simulink model "motorSimIdent"  (R2019b)
settings: Solver=VariableStepAuto  StartTime=0.0  StopTime=10.0  RelTol=1e-3
values from neighbouring files (symbols this model uses):
  b = 0.5    [MotorExpScriptIdent.m]    (also in motorSimScript.m; motorSimScriptIdent.m)
  J = 0.05    [MotorExpScriptIdent.m]    (also in motorSimScript.m; motorSimScriptIdent.m)
  K = 114.4795944    [MotorExpScriptIdent.m]    (also in motorSimScript.m = 8; motorSimScriptIdent.m = 10)
  Ke = 0.5    [MotorExpScriptIdent.m]    (also in motorSimScript.m; motorSimScriptIdent.m)
  Kt = 0.5    [MotorExpScriptIdent.m]    (also in motorSimScript.m; motorSimScriptIdent.m)
  Ra = 1    [MotorExpScriptIdent.m]    (also in motorSimScript.m; motorSimScriptIdent.m)
  sigma = 0.1147802808    [MotorExpScriptIdent.m]    (also in motorSimScript.m = 0.2; motorSimScriptIdent.m = 0.2)
settings Model: Creator=coffe  LastModifiedBy=coffe

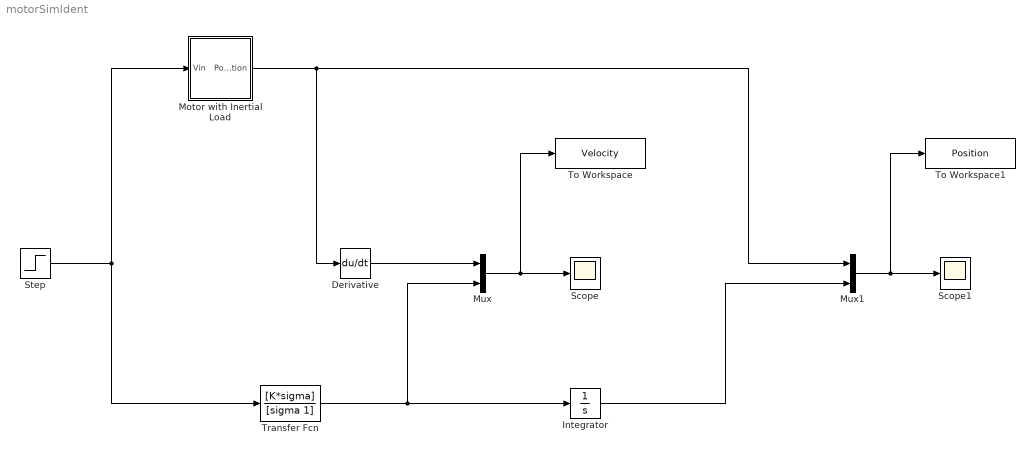
== system motorSimIdent ==
  Derivative : Derivative
  Integrator : Integrator
  Motor with Inertial Load : Subsystem
  Mux : Mux  Inputs=2
  Mux1 : Mux  Inputs=2
  Scope : Scope
  Scope1 : Scope
  Step : Step  SampleTime=0
  To Workspace : ToWorkspace  VariableName=Velocity  SaveFormat=Timeseries  SampleTime=-1
  To Workspace1 : ToWorkspace  VariableName=Position  SaveFormat=Timeseries  SampleTime=-1
  Transfer Fcn : TransferFcn  Numerator=[K*sigma]  Denominator=[sigma 1]
  wires:
  Mux/1 -> Scope/1, To Workspace/1
  Motor with Inertial Load/1(Position) -> Mux1/1, Derivative/1
  Mux1/1 -> Scope1/1, To Workspace1/1
  Step/1 -> Transfer Fcn/1, Motor with Inertial Load/1(Vin)
  Derivative/1 -> Mux/1
  Integrator/1 -> Mux1/2
  Transfer Fcn/1 -> Mux/2, Integrator/1

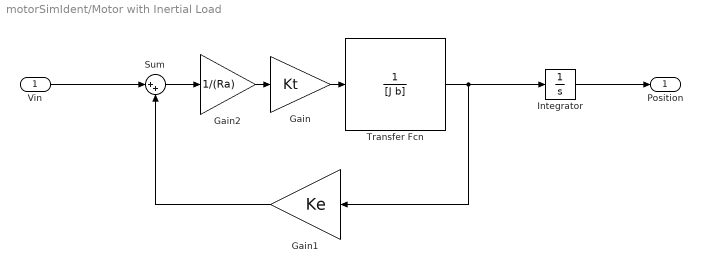
== system motorSimIdent/Motor with Inertial Load ==
  Vin : Inport
  Gain : Gain  Gain=Kt
  Gain1 : Gain  Gain=Ke
  Gain2 : Gain  Gain=1/(Ra)
  Integrator : Integrator
  Sum : Sum  Inputs=|++
  Transfer Fcn : TransferFcn  Denominator=[J b]
  Position : Outport
  wires:
  Gain/1 -> Transfer Fcn/1
  Transfer Fcn/1 -> Integrator/1, Gain1/1
  Gain2/1 -> Gain/1
  Vin/1 -> Sum/1
  Gain1/1 -> Sum/2
  Sum/1 -> Gain2/1
  Integrator/1 -> Position/1
